simulink model "BuckyWagon_01"  (Simulink 7.5)
settings: Solver=FixedStepDiscrete  StartTime=0.0  StopTime=10.0  RelTol=1e-3
PreLoadFcn:
  | try, eval([bdroot '_setup']); catch, eval('model_setup', ''); end
InitFcn:
  | try, eval([bdroot '_setup']); catch, eval('model_setup', ''); end
undefined symbols (not defined in the file): ECU565, High, Low, miniviewSetup, motohawk_build_version, motohawk_get_faults, motohawk_setup_toolchains, motohawk_trunc_name, motohawk_vardec_config_group, motohawk_vardec_path, tc, True
libraries: MotoHawk_lib x499, simulink x29, motohawk_engine_lib x19, miniview_lib x10, motohawk_control_primitives_lib x8, motohawk_annotations_lib x2
(part 7 of 9)

== system BuckyWagon_01/Strategy/MiniViewDisplay/GetFaultName ==
  Chart : Stateflow chart  TreatAsAtomicUnit=on
  Fault Iterator : Subsystem  TreatAsAtomicUnit=on
  Unit Delay : UnitDelay  SampleTime=-1
  Unit Delay1 : UnitDelay  SampleTime=-1
  getStringLength : Stateflow chart  TreatAsAtomicUnit=on
  motohawk_calibration : MotoHawk_lib/Calibration & Probing Blocks/motohawk_calibration  nam='DisplayFaults'  val=0  storage=Calibration  show_more=on  name_source=Use Parameter  data_type=boolean  read_level=1  write_level=1  ovr_cals=on  view_as=Enumeration  enum_struct={'Disabled', 'Enabled'}  vector_style=Wide Row  use_help_units=on  help='Enable displaying faults when they are active.'  units=''  use_header_enum=off  row_header_enum={}  col_header_enum={}  use_min_max=off  min_val=-inf  max_val=inf  use_precision=off  precision=''  gain=1  offset=0  exp=1  use_mototune_group=off  mototune_group=motohawk_vardec_path(gcb)
  motohawk_calibration1 : MotoHawk_lib/Calibration & Probing Blocks/motohawk_calibration  nam='InvertMode'  val=0  storage=Calibration  show_more=on  name_source=Use Parameter  data_type=boolean  read_level=1  write_level=1  ovr_cals=on  view_as=Enumeration  enum_struct={'Normal', 'Inverted'}  vector_style=Wide Row  use_help_units=on  help='Sets the background color for the text.'  units=''  use_header_enum=off  row_header_enum={}  col_header_enum={}  use_min_max=off  min_val=-inf  max_val=inf  use_precision=off  precision=''  gain=1  offset=0  exp=1  use_mototune_group=off  mototune_group=motohawk_vardec_path(gcb)
  motohawk_calibration2 : MotoHawk_lib/Calibration & Probing Blocks/motohawk_calibration  nam='noErrText'  val=[uint8(' BuckEV') 0 0 0]  storage=Calibration  show_more=on  name_source=Use Parameter  data_type=uint8  read_level=1  write_level=1  ovr_cals=on  view_as=Text  enum_struct={'Disabled', 'Enabled'}  vector_style=Wide Row  use_help_units=on  help='Text to display if there are no faults.'  units=''  use_header_enum=off  row_header_enum={}  col_header_enum={}  use_min_max=off  min_val=-inf  max_val=inf  use_precision=off  precision=''  gain=1  offset=0  exp=1  use_mototune_group=off  mototune_group=motohawk_vardec_path(gcb)
  motohawk_calibration3 : MotoHawk_lib/Calibration & Probing Blocks/motohawk_calibration  nam='dispLength'  val=7  storage=Calibration  show_more=on  name_source=Use Parameter  data_type=uint8  read_level=1  write_level=1  ovr_cals=on  view_as=Number  enum_struct={'Disabled', 'Enabled'}  vector_style=Wide Row  use_help_units=on  help='Number of characters to display when scrolling fault name.'  units=''  use_header_enum=off  row_header_enum={}  col_header_enum={}  use_min_max=on  min_val=0  max_val=9  use_precision=on  precision=''  gain=1  offset=0  exp=1  use_mototune_group=off  mototune_group=motohawk_vardec_path(gcb)
  motohawk_calibration4 : MotoHawk_lib/Calibration & Probing Blocks/motohawk_calibration  nam='lastScrollTime'  val=1/0.005  storage=Calibration  show_more=on  name_source=Use Parameter  data_type=uint16  read_level=1  write_level=1  ovr_cals=on  view_as=Number  enum_struct={'Disabled', 'Enabled'}  vector_style=Wide Row  use_help_units=on  help='Time to spend on the last view of the scroll'  units='s'  use_header_enum=off  row_header_enum={}  col_header_enum={}  use_min_max=on  min_val=0  max_val=5  use_precision=on  precision='1.3'  gain=0.005  offset=0  exp=1  use_mototune_group=off  mototune_group=motohawk_vardec_path(gcb)
  motohawk_calibration5 : MotoHawk_lib/Calibration & Probing Blocks/motohawk_calibration  nam='scrollTime'  val=0.6/0.005  storage=Calibration  show_more=on  name_source=Use Parameter  data_type=uint16  read_level=1  write_level=1  ovr_cals=on  view_as=Number  enum_struct={'Disabled', 'Enabled'}  vector_style=Wide Row  use_help_units=on  help='Time to spend on each view of the scroll'  units='s'  use_header_enum=off  row_header_enum={}  col_header_enum={}  use_min_max=on  min_val=0  max_val=5  use_precision=on  precision='1.3'  gain=0.005  offset=0  exp=1  use_mototune_group=off  mototune_group=motohawk_vardec_path(gcb)
  motohawk_calibration6 : MotoHawk_lib/Calibration & Probing Blocks/motohawk_calibration  nam='minTime'  val=3/0.005  storage=Calibration  show_more=on  name_source=Use Parameter  data_type=uint16  read_level=1  write_level=1  ovr_cals=on  view_as=Number  enum_struct={'Disabled', 'Enabled'}  vector_style=Wide Row  use_help_units=on  help='Minimum time to display each fault name.'  units='s'  use_header_enum=off  row_header_enum={}  col_header_enum={}  use_min_max=on  min_val=0  max_val=5  use_precision=on  precision='1.3'  gain=0.005  offset=0  exp=1  use_mototune_group=off  mototune_group=motohawk_vardec_path(gcb)
  motohawk_calibration7 : MotoHawk_lib/Calibration & Probing Blocks/motohawk_calibration  nam='firstScrollTime'  val=1/0.005  storage=Calibration  show_more=on  name_source=Use Parameter  data_type=uint16  read_level=1  write_level=1  ovr_cals=on  view_as=Number  enum_struct={'Disabled', 'Enabled'}  vector_style=Wide Row  use_help_units=on  help='Time to spend on first view of the scroll'  units='s'  use_header_enum=off  row_header_enum={}  col_header_enum={}  use_min_max=on  min_val=0  max_val=5  use_precision=on  precision='1.3'  gain=0.005  offset=0  exp=1  use_mototune_group=off  mototune_group=motohawk_vardec_path(gcb)
  motohawk_probe : MotoHawk_lib/Calibration & Probing Blocks/motohawk_probe  nam='minTimer'  show_more=on  name_source=Use Parameter  read_level=1  view_as=Number  enum_struct={'Disabled', 'Enabled'}  vector_style=Wide Row  use_help_units=off  help=''  units=''  use_header_enum=off  row_header_enum={}  col_header_enum={}  use_precision=on  precision='1.3'  gain=0.005  offset=0  exp=1  use_mototune_group=off  mototune_group=motohawk_vardec_path(gcb)
  motohawk_probe2 : MotoHawk_lib/Calibration & Probing Blocks/motohawk_probe  nam='scrollTimer'  show_more=on  name_source=Use Parameter  read_level=1  view_as=Number  enum_struct={'Disabled', 'Enabled'}  vector_style=Wide Row  use_help_units=off  help=''  units=''  use_header_enum=off  row_header_enum={}  col_header_enum={}  use_precision=on  precision='1.3'  gain=0.005  offset=0  exp=1  use_mototune_group=off  mototune_group=motohawk_vardec_path(gcb)
  motohawk_probe3 : MotoHawk_lib/Calibration & Probing Blocks/motohawk_probe  nam='scrollIndex'  show_more=off  name_source=Use Parameter  read_level=1  view_as=Number  enum_struct={'Disabled', 'Enabled'}  vector_style=Wide Row  use_help_units=off  help=''  units=''  use_header_enum=off  row_header_enum={}  col_header_enum={}  use_precision=off  precision=''  gain=1  offset=0  exp=1  use_mototune_group=off  mototune_group=motohawk_vardec_path(gcb)
  Name : Outport  OutDataType=sfix(16)  OutScaling=2^0
  Mode : Outport  Port=2  OutDataType=sfix(16)  OutScaling=2^0
  wires:
  Chart/6(getNewFault) -> Fault Iterator/Trigger
  Chart/2(text) -> Name/1
  Chart/1(mode) -> Mode/1
  Chart/3(minTimer) -> motohawk_probe/1
  Chart/4(scrollIndex) -> motohawk_probe3/1
  Chart/5(scrollTimer) -> motohawk_probe2/1
  motohawk_calibration/1 -> Chart/7(dispFaults)
  motohawk_calibration1/1 -> Chart/1(invertMode)
  motohawk_calibration2/1 -> Chart/2(noErrText)
  motohawk_calibration3/1 -> Chart/3(dispLength)
  Fault Iterator/2(valid) -> Unit Delay1/1
  Fault Iterator/1(Name) -> Unit Delay/1
  motohawk_calibration4/1 -> Chart/4(lastScrollTime)
  motohawk_calibration5/1 -> Chart/5(scrollTime)
  motohawk_calibration6/1 -> Chart/8(minTime)
  getStringLength/1(faultNameLength) -> Chart/9(faultNameLen)
  Unit Delay/1 -> Chart/10(faultName), getStringLength/1(faultName)
  Unit Delay1/1 -> Chart/11(faultValid)
  motohawk_calibration7/1 -> Chart/6(firstScrollTime)

== system BuckyWagon_01/Strategy/MiniViewDisplay/Menu Button ==
  CAN Receive Slot Trigger : MotoHawk_lib/CAN Blocks/CAN Receive Slot Trigger  Tag=Trigger  slot='miniview_button_menu'  inherited=on  function_name=Trigger_CAN_Slot_miniview_button_menu_2154p0004
  Demux : Demux  Outputs=2
  Subsystem : Subsystem
  Update : Outport  OutDataType=sfix(16)  OutScaling=2^0
  Menu Asserted : Outport  Port=2  OutDataType=sfix(16)  OutScaling=2^0
  Menu Count : Outport  Port=3  OutDataType=sfix(16)  OutScaling=2^0
  wires:
  Subsystem/1(Out1) -> Menu Asserted/1
  Demux/1 -> Subsystem/Trigger
  CAN Receive Slot Trigger/1 -> Demux/1
  Demux/2 -> Update/1
  Subsystem/2(Out2) -> Menu Count/1

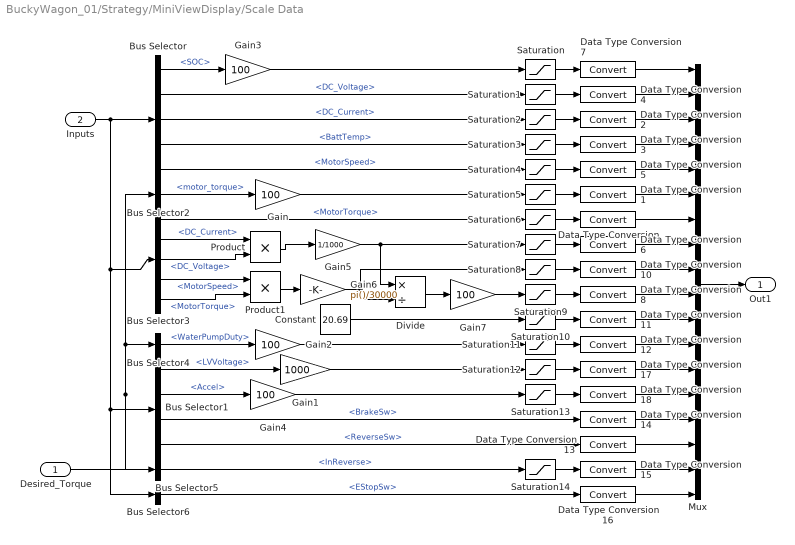
== system BuckyWagon_01/Strategy/MiniViewDisplay/Scale Data ==
  Desired_Torque : Inport  OutDataType=sfix(16)  OutScaling=2^0
  Inputs : Inport  Port=2  OutDataType=sfix(16)  OutScaling=2^0
  Bus Selector : BusSelector  OutputSignals=Virtual.SOC,Physical.DC_Voltage,Physical.DC_Current,Physical.BattTemp,Physical.MotorSpeed
  Bus Selector1 : BusSelector  OutputSignals=Physical.LVVoltage,Physical.Accel,Physical.BrakeSw,Physical.ReverseSw
  Bus Selector2 : BusSelector  OutputSignals=motor_torque
  Bus Selector3 : BusSelector  OutputSignals=Physical.MotorTorque,Physical.DC_Current,Physical.DC_Voltage,Physical.MotorSpeed,Physical.MotorTorque
  Bus Selector4 : BusSelector  OutputSignals=WaterPumpDuty
  Bus Selector5 : BusSelector  OutputSignals=InReverse
  Bus Selector6 : BusSelector  OutputSignals=Physical.EStopSw
  Constant : Constant  Value=20.69  OutDataType=fixdt(1, 16)  OutScaling=2^0
  Data Type Conversion{,1..8,10..18} (18 alike) : DataTypeConversion  OutDataType=sfix(16)  OutScaling=2^0
  Divide : Product  Inputs=*/  OutDataType=sfix(16)  OutScaling=2^-10
  Gain{,2..4,7} (5 alike) : Gain  Gain=100  ParameterDataType=sfix(16)  ParameterScaling=2^0  OutDataType=sfix(16)  OutScaling=2^0  OutDataTypeStr=Inherit: Inherit via back propagation
  Gain1 : Gain  Gain=1000  ParameterDataType=sfix(16)  ParameterScaling=2^0  OutDataType=sfix(16)  OutScaling=2^0  OutDataTypeStr=Inherit: Inherit via back propagation
  Gain5 : Gain  Gain=1/1000  ParameterDataType=sfix(16)  ParameterScaling=2^0  OutDataType=sfix(16)  OutScaling=2^0  OutDataTypeStr=Inherit: Inherit via back propagation
  Gain6 : Gain  Gain=pi()/30000  ParameterDataType=sfix(16)  ParameterScaling=2^0  OutDataType=sfix(16)  OutScaling=2^0  OutDataTypeStr=Inherit: Inherit via back propagation
  Mux : Mux  Inputs=18
  Product : Product  OutDataType=sfix(16)  OutScaling=2^0  RndMeth=Zero
  Product1 : Product  OutDataType=sfix(16)  OutScaling=2^0  RndMeth=Zero
  Saturation{,1..8,10..14} (14 alike) : Saturate  UpperLimit=32767  LowerLimit=-32767  OutDataType=sfix(16)  OutScaling=2^0
  Saturation9 : Saturate  UpperLimit=100  LowerLimit=0  OutDataType=sfix(16)  OutScaling=2^0
  Out1 : Outport  OutDataType=sfix(16)  OutScaling=2^0
  wires:
  Desired_Torque/1 -> Bus Selector2/1, Bus Selector4/1, Bus Selector5/1
  Bus Selector/3 -> Saturation2/1  "<DC_Current>"
  Bus Selector/4 -> Saturation3/1  "<BattTemp>"
  Bus Selector/2 -> Saturation1/1  "<DC_Voltage>"
  Bus Selector/5 -> Saturation4/1  "<MotorSpeed>"
  Bus Selector/1 -> Gain3/1  "<SOC>"
  Mux/1 -> Out1/1
  Gain3/1 -> Saturation/1
  Data Type Conversion4/1 -> Mux/2
  Data Type Conversion2/1 -> Mux/3
  Data Type Conversion3/1 -> Mux/4
  Data Type Conversion5/1 -> Mux/5
  Gain/1 -> Saturation5/1
  Bus Selector2/1 -> Gain/1  "<motor_torque>"
  Inputs/1 -> Bus Selector/1, Bus Selector3/1, Bus Selector1/1, Bus Selector6/1
  Bus Selector3/1 -> Saturation6/1  "<MotorTorque>"
  Bus Selector3/2 -> Product/1  "<DC_Current>"
  Bus Selector3/3 -> Product/2  "<DC_Voltage>"
  Product/1 -> Gain5/1
  Bus Selector3/4 -> Product1/1  "<MotorSpeed>"
  Bus Selector3/5 -> Product1/2  "<MotorTorque>"
  Product1/1 -> Gain6/1
  Constant/1 -> Saturation10/1
  Gain5/1 -> Divide/1, Saturation7/1
  Gain6/1 -> Divide/2, Saturation8/1
  Data Type Conversion/1 -> Mux/7
  Divide/1 -> Gain7/1
  Gain7/1 -> Saturation9/1
  Data Type Conversion6/1 -> Mux/8
  Data Type Conversion10/1 -> Mux/9
  Bus Selector4/1 -> Gain2/1  "<WaterPumpDuty>"
  Gain2/1 -> Saturation11/1
  Bus Selector1/1 -> Gain1/1  "<LVVoltage>"
  Bus Selector1/2 -> Gain4/1  "<Accel>"
  Bus Selector1/3 -> Data Type Conversion14/1  "<BrakeSw>"
  Bus Selector1/4 -> Data Type Conversion13/1  "<ReverseSw>"
  Gain1/1 -> Saturation12/1
  Gain4/1 -> Saturation13/1
  Data Type Conversion14/1 -> Mux/15
  Data Type Conversion13/1 -> Mux/16
  Bus Selector5/1 -> Saturation14/1  "<InReverse>"
  Data Type Conversion15/1 -> Mux/17
  Bus Selector6/1 -> Data Type Conversion16/1  "<EStopSw>"
  Data Type Conversion16/1 -> Mux/18
  Data Type Conversion1/1 -> Mux/6
  Data Type Conversion7/1 -> Mux/1
  Data Type Conversion8/1 -> Mux/10
  Data Type Conversion11/1 -> Mux/11
  Data Type Conversion12/1 -> Mux/12
  Data Type Conversion17/1 -> Mux/13
  Data Type Conversion18/1 -> Mux/14
  Saturation/1 -> Data Type Conversion7/1
  Saturation1/1 -> Data Type Conversion4/1
  Saturation2/1 -> Data Type Conversion2/1
  Saturation3/1 -> Data Type Conversion3/1
  Saturation4/1 -> Data Type Conversion5/1
  Saturation5/1 -> Data Type Conversion1/1
  Saturation6/1 -> Data Type Conversion/1
  Saturation7/1 -> Data Type Conversion6/1
  Saturation8/1 -> Data Type Conversion10/1
  Saturation9/1 -> Data Type Conversion8/1
  Saturation10/1 -> Data Type Conversion11/1
  Saturation11/1 -> Data Type Conversion12/1
  Saturation12/1 -> Data Type Conversion17/1
  Saturation13/1 -> Data Type Conversion18/1
  Saturation14/1 -> Data Type Conversion15/1

== system BuckyWagon_01/Strategy/MiniViewDisplay/Send String_efficient ==
  string # : Inport  OutDataType=sfix(16)  OutScaling=2^0
  string : Inport  Port=2  OutDataType=sfix(16)  OutScaling=2^0
  Trigger : TriggerPort  TriggerType=function-call
  Demux : Demux  Outputs=2
  Function-Call Generator : simulink/Ports & Subsystems/Function-Call Generator  sample_time=-1  numberOfIterations=1
  Signal Specification : SignalSpecification  Dimensions=18  DataType=uint8  OutDataType=sfix(16)  OutScaling=2^0  OutDataTypeStr=uint8
  Subsystem : Subsystem
  Next : Outport  OutDataType=sfix(16)  OutScaling=2^0
  wires:
  Signal Specification/1 -> Subsystem/2(string)
  Demux/2 -> Next/1
  Function-Call Generator/1 -> Demux/1
  Demux/1 -> Subsystem/Trigger
  string/1 -> Signal Specification/1  "b0"
  string #/1 -> Subsystem/1(string #)  "string"

== system BuckyWagon_01/Strategy/MiniViewDisplay/Up Button ==
  CAN Receive Slot Trigger : MotoHawk_lib/CAN Blocks/CAN Receive Slot Trigger  Tag=Trigger  slot='miniview_button_up'  inherited=on  function_name=Trigger_CAN_Slot_miniview_button_up_2402p0004
  Demux : Demux  Outputs=2
  Subsystem : Subsystem
  Update : Outport  OutDataType=sfix(16)  OutScaling=2^0
  Up Asserted : Outport  Port=2  OutDataType=sfix(16)  OutScaling=2^0
  Up Count : Outport  Port=3  OutDataType=sfix(16)  OutScaling=2^0
  wires:
  Subsystem/2(Up Count) -> Up Count/1
  Demux/2 -> Update/1
  CAN Receive Slot Trigger/1 -> Demux/1
  Demux/1 -> Subsystem/Trigger
  Subsystem/1(Up Asserted) -> Up Asserted/1

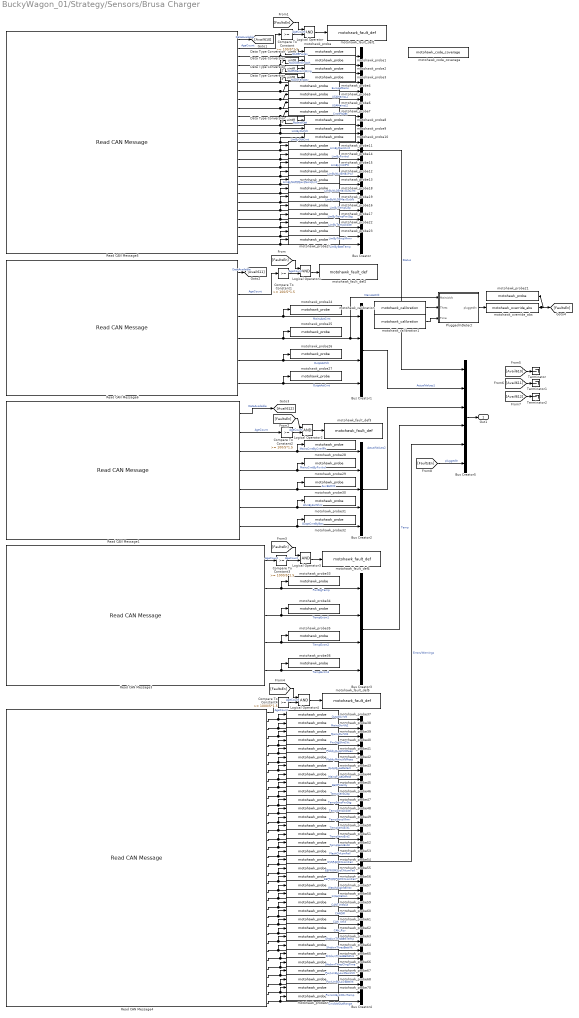
== system BuckyWagon_01/Strategy/Sensors/Brusa Charger ==
  Bus Creator : BusCreator  Inputs=23
  Bus Creator1 : BusCreator
  Bus Creator2 : BusCreator  Inputs=5
  Bus Creator3 : BusCreator
  Bus Creator4 : BusCreator  Inputs=34
  Bus Creator5 : BusCreator  Inputs=6
  Compare To Constant : simulink/Logic and Bit Operations/Compare To Constant  SystemSampleTime=-1  relop=>=  const=100/5*1.5  LogicOutDataTypeMode=boolean  ZeroCross=off
  Compare To Constant1 : simulink/Logic and Bit Operations/Compare To Constant  SystemSampleTime=-1  relop=>=  const=100/5*1.5  LogicOutDataTypeMode=boolean  ZeroCross=off
  Compare To Constant2 : simulink/Logic and Bit Operations/Compare To Constant  SystemSampleTime=-1  relop=>=  const=100/5*1.5  LogicOutDataTypeMode=boolean  ZeroCross=off
  Compare To Constant3 : simulink/Logic and Bit Operations/Compare To Constant  SystemSampleTime=-1  relop=>=  const=1000/5*1.5  LogicOutDataTypeMode=boolean  ZeroCross=off
  Compare To Constant4 : simulink/Logic and Bit Operations/Compare To Constant  SystemSampleTime=-1  relop=>=  const=1000/5*1.5  LogicOutDataTypeMode=boolean  ZeroCross=off
  Data Type Conversion{,1..4} (5 alike) : DataTypeConversion  OutDataTypeMode=uint8  OutDataType=sfix(16)  OutScaling=2^0  OutDataTypeStr=uint8
  Logical Operator{,1..4} (5 alike) : Logic  AllPortsSameDT=off  OutDataTypeMode=boolean  OutDataTypeStr=boolean
  PluggedInDetect : Subsystem
  Read CAN Message1 : MotoHawk_lib/CAN Blocks/Read CAN Message  nam=['CAN_' num2str(1)]  bus=-2  msg=can_BRUSA_612  queue=1  slot=''  valid=on  stale=on  labelwires=on
  Read CAN Message3 : MotoHawk_lib/CAN Blocks/Read CAN Message  nam=['CAN_' num2str(1)]  bus=-2  msg=can_BRUSA_613  queue=1  slot=''  valid=off  stale=on  labelwires=on
  Read CAN Message4 : MotoHawk_lib/CAN Blocks/Read CAN Message  nam=['CAN_' num2str(1)]  bus=-2  msg=can_BRUSA_614  queue=1  slot=''  valid=off  stale=on  labelwires=on
  Read CAN Message5 : MotoHawk_lib/CAN Blocks/Read CAN Message  nam=['CAN_' num2str(1)]  bus=-2  msg=can_BRUSA_610  queue=1  slot=''  valid=on  stale=on  labelwires=on
  Read CAN Message6 : MotoHawk_lib/CAN Blocks/Read CAN Message  nam=['CAN_' num2str(1)]  bus=-2  msg=can_BRUSA_611  queue=1  slot=''  valid=on  stale=on  labelwires=on
  Terminator : Terminator
  Terminator1 : Terminator
  Terminator2 : Terminator
  motohawk_calibration : MotoHawk_lib/Calibration & Probing Blocks/motohawk_calibration  nam='PluggedInMainsThes'  val=90  storage=Calibration  show_more=on  name_source=Use Parameter  data_type=Inherit from 'Default Value'  read_level=1  write_level=1  ovr_cals=on  view_as=Number  enum_struct={'Disabled', 'Enabled'}  vector_style=Wide Row  use_help_units=on  help='Above this mains voltage the charger is plugged in.'  units='V'  use_header_enum=off  row_header_enum={}  col_header_enum={}  use_min_max=off  min_val=-inf  max_val=inf  use_precision=off  precision=''  gain=1  offset=0  exp=1  use_mototune_group=off  mototune_group=motohawk_vardec_path(gcb)
  motohawk_calibration1 : MotoHawk_lib/Calibration & Probing Blocks/motohawk_calibration  nam='PluggedInHistTime'  val=0.5/0.005  storage=Calibration  show_more=on  name_source=Use Parameter  data_type=Inherit from 'Default Value'  read_level=1  write_level=1  ovr_cals=on  view_as=Number  enum_struct={'Disabled', 'Enabled'}  vector_style=Wide Row  use_help_units=on  help='Historesis time for plugged in detection.'  units='s'  use_header_enum=off  row_header_enum={}  col_header_enum={}  use_min_max=off  min_val=-inf  max_val=inf  use_precision=on  precision='1.2'  gain=0.005  offset=0  exp=1  use_mototune_group=off  mototune_group=motohawk_vardec_path(gcb)
  motohawk_code_coverage : MotoHawk_lib/Extra Development Blocks/motohawk_code_coverage
  motohawk_fault_def1 : MotoHawk_lib/Fault Management Blocks/motohawk_fault_def  nam='canNLG5_610'  mode=Enabled  id=[]  x=100/5*0.5  y=100/5*2  input_suspected=on  indeterminate=off  increment_xy=on  downsample_count=1  ovr_cals=on  ovr_actions=on  show_actions=on  action1_name='Charge_Fault'  action1_cond=Active  action2_name=''  action2_cond=(None)  action3_name=''  action3_cond=(None)  action4_name=''  action4_cond=(None)
  motohawk_fault_def2 : MotoHawk_lib/Fault Management Blocks/motohawk_fault_def  nam='canNLG5_611'  mode=Enabled  id=[]  x=100/5*0.5  y=100/5*2  input_suspected=on  indeterminate=off  increment_xy=on  downsample_count=1  ovr_cals=on  ovr_actions=on  show_actions=on  action1_name='Charge_Fault'  action1_cond=Active  action2_name=''  action2_cond=(None)  action3_name=''  action3_cond=(None)  action4_name=''  action4_cond=(None)
  motohawk_fault_def3 : MotoHawk_lib/Fault Management Blocks/motohawk_fault_def  nam='canNLG5_612'  mode=Enabled  id=[]  x=100/5*0.5  y=100/5*2  input_suspected=on  indeterminate=off  increment_xy=on  downsample_count=1  ovr_cals=on  ovr_actions=on  show_actions=on  action1_name='Charge_Fault'  action1_cond=(None)  action2_name=''  action2_cond=(None)  action3_name=''  action3_cond=(None)  action4_name=''  action4_cond=(None)
  motohawk_fault_def4 : MotoHawk_lib/Fault Management Blocks/motohawk_fault_def  nam='canNLG5_613'  mode=Enabled  id=[]  x=1000/5*0.5  y=1000/5*2  input_suspected=on  indeterminate=off  increment_xy=on  downsample_count=1  ovr_cals=on  ovr_actions=on  show_actions=off  action1_name=''  action1_cond=(None)  action2_name=''  action2_cond=(None)  action3_name=''  action3_cond=(None)  action4_name=''  action4_cond=(None)
  motohawk_fault_def5 : MotoHawk_lib/Fault Management Blocks/motohawk_fault_def  nam='canNLG5_614'  mode=Enabled  id=[]  x=1000/5*0.5  y=1000/5*2  input_suspected=on  indeterminate=off  increment_xy=on  downsample_count=1  ovr_cals=on  ovr_actions=on  show_actions=off  action1_name=''  action1_cond=(None)  action2_name=''  action2_cond=(None)  action3_name=''  action3_cond=(None)  action4_name=''  action4_cond=(None)
  motohawk_override_abs : MotoHawk_lib/Calibration & Probing Blocks/motohawk_override_abs  SystemSampleTime=-1  parent_name='pluggedIn'  parent_val=0  show_more=off  name_source=Use Parameter  parent_read_level=1  parent_override_level=1  view_as=Number  enum_struct={'Disabled', 'Enabled'}  use_help_units=off  parent_help=''  parent_units=''  use_min_max=off  parent_min=-inf  parent_max=inf  use_precision=off  parent_precision=''  parent_gain=1  parent_offset=0  parent_exp=1  use_mototune_group=off  parent_group=motohawk_vardec_path(gcb)
  motohawk_probe : MotoHawk_lib/Calibration & Probing Blocks/motohawk_probe  nam='NLG5PwrEn'  show_more=on  name_source=Use Parameter  read_level=1  view_as=Enumeration  enum_struct={'Disabled', 'Enabled'}  vector_style=Wide Row  use_help_units=off  help=''  units=''  use_header_enum=off  row_header_enum={}  col_header_enum={}  use_precision=off  precision=''  gain=1  offset=0  exp=1  use_mototune_group=off  mototune_group=motohawk_vardec_path(gcb)
  motohawk_probe1 : MotoHawk_lib/Calibration & Probing Blocks/motohawk_probe  nam='NLG5GenErrLtch'  show_more=on  name_source=Use Parameter  read_level=1  view_as=Enumeration  enum_struct={'No Error', 'ERROR'}  vector_style=Wide Row  use_help_units=off  help=''  units=''  use_header_enum=off  row_header_enum={}  col_header_enum={}  use_precision=off  precision=''  gain=1  offset=0  exp=1  use_mototune_group=off  mototune_group=motohawk_vardec_path(gcb)
  motohawk_probe{4..7,9..20,22..70} (65 alike) : MotoHawk_lib/Calibration & Probing Blocks/motohawk_probe  nam='Probe'  show_more=on  name_source=Use Input Wire Name  read_level=1  view_as=Number  enum_struct={'Disabled', 'Enabled'}  vector_style=Wide Row  use_help_units=off  help=''  units=''  use_header_enum=off  row_header_enum={}  col_header_enum={}  use_precision=off  precision=''  gain=1  offset=0  exp=1  use_mototune_group=off  mototune_group=motohawk_vardec_path(gcb)
  motohawk_probe2 : MotoHawk_lib/Calibration & Probing Blocks/motohawk_probe  nam='NLG5GenLimWrng'  show_more=on  name_source=Use Parameter  read_level=1  view_as=Enumeration  enum_struct={'No Warn', 'WARNING'}  vector_style=Wide Row  use_help_units=off  help=''  units=''  use_header_enum=off  row_header_enum={}  col_header_enum={}  use_precision=off  precision=''  gain=1  offset=0  exp=1  use_mototune_group=off  mototune_group=motohawk_vardec_path(gcb)
  motohawk_probe21 : MotoHawk_lib/Calibration & Probing Blocks/motohawk_probe  nam='pluggedIn'  show_more=off  name_source=Use Parameter  read_level=1  view_as=Number  enum_struct={'Disabled', 'Enabled'}  vector_style=Wide Row  use_help_units=off  help=''  units=''  use_header_enum=off  row_header_enum={}  col_header_enum={}  use_precision=off  precision=''  gain=1  offset=0  exp=1  use_mototune_group=off  mototune_group=motohawk_vardec_path(gcb)
  motohawk_probe3 : MotoHawk_lib/Calibration & Probing Blocks/motohawk_probe  nam='NLG5FanActv'  show_more=on  name_source=Use Parameter  read_level=1  view_as=Enumeration  enum_struct={'Off', 'On'}  vector_style=Wide Row  use_help_units=off  help=''  units=''  use_header_enum=off  row_header_enum={}  col_header_enum={}  use_precision=off  precision=''  gain=1  offset=0  exp=1  use_mototune_group=off  mototune_group=motohawk_vardec_path(gcb)
  motohawk_probe8 : MotoHawk_lib/Calibration & Probing Blocks/motohawk_probe  nam='BypassDet'  show_more=on  name_source=Use Parameter  read_level=1  view_as=Enumeration  enum_struct={'none', 'DC', 'AC in Phase', 'AC not in Phase'}  vector_style=Wide Row  use_help_units=off  help=''  units=''  use_header_enum=off  row_header_enum={}  col_header_enum={}  use_precision=off  precision=''  gain=1  offset=0  exp=1  use_mototune_group=off  mototune_group=motohawk_vardec_path(gcb)
  Out1 : Outport  OutDataType=sfix(16)  OutScaling=2^0
  wires:
  Read CAN Message5/2 -> Compare To Constant/1  "AgeCount"
  Read CAN Message5/3 -> Bus Creator/1, Data Type Conversion/1  "NLG5PwrEn"
  Read CAN Message5/4 -> Bus Creator/2, Data Type Conversion1/1  "NLG5GenErrLtch"
  Read CAN Message5/5 -> Bus Creator/3, Data Type Conversion2/1  "NLG5GenLimWrng"
  Read CAN Message5/6 -> Bus Creator/4, Data Type Conversion3/1  "NLG5FanActv"
  Read CAN Message5/7 -> Bus Creator/5, motohawk_probe4/1  "EuropeMains"
  Read CAN Message5/8 -> Bus Creator/6, motohawk_probe5/1  "USAMainsL1"
  Read CAN Message5/9 -> Bus Creator/7, motohawk_probe6/1  "USAMainsL2"
  Read CAN Message5/10 -> Bus Creator/8, motohawk_probe7/1  "CntrlPltDet"
  Read CAN Message5/11 -> Bus Creator/9, Data Type Conversion4/1  "BypassDet"
  Read CAN Message5/12 -> Bus Creator/10, motohawk_probe9/1  "LimByOutVlt"
  Read CAN Message5/13 -> Bus Creator/11, motohawk_probe10/1  "LimByOutCrnt"
  Read CAN Message5/14 -> Bus Creator/12, motohawk_probe11/1  "LimByMainCrnt"
  Read CAN Message5/15 -> Bus Creator/13, motohawk_probe14/1  "LimByPwrInd"
  Read CAN Message5/16 -> Bus Creator/14, motohawk_probe15/1  "LimByCntrlPlt"
  Read CAN Message5/17 -> Bus Creator/15, motohawk_probe12/1  "LimByNLG5MaxPwr"
  Read CAN Message5/18 -> Bus Creator/16, motohawk_probe13/1  "LimByNLG5MaxMainsCrnt"
  Read CAN Message5/19 -> Bus Creator/17, motohawk_probe18/1  "LimByNLG5MaxOutCrnt"
  Read CAN Message5/20 -> Bus Creator/18, motohawk_probe19/1  "LimByNLG5MaxOutVlt"
  Read CAN Message5/21 -> Bus Creator/19, motohawk_probe16/1  "LimByTempCap"
  Read CAN Message5/22 -> Bus Creator/20, motohawk_probe17/1  "LimByTempPwrStg"
  Read CAN Message5/23 -> Bus Creator/21, motohawk_probe22/1  "LimByTempDiode"
  Read CAN Message5/24 -> Bus Creator/22, motohawk_probe23/1  "LimByTempXfrmr"
  Read CAN Message5/25 -> Bus Creator/23, motohawk_probe20/1  "LimByBattTemp"
  Read CAN Message1/3 -> motohawk_probe28/1, Bus Creator2/1  "MainsCrntByCntrlPlt"
  Read CAN Message1/4 -> motohawk_probe29/1, Bus Creator2/2  "MainsCrntByPwrInd"
  Read CAN Message1/5 -> motohawk_probe30/1, Bus Creator2/3  "AuxBattVlt"
  Read CAN Message1/6 -> motohawk_probe31/1, Bus Creator2/4  "AhrsByExtShnt"
  Read CAN Message1/7 -> Bus Creator2/5, motohawk_probe32/1  "OutptCrntByBstr"
  Read CAN Message1/2 -> Compare To Constant2/1  "AgeCount"
  Read CAN Message6/3 -> Bus Creator1/1, motohawk_probe24/1  "MainsActCrnt"
  Read CAN Message6/4 -> motohawk_probe25/1, Bus Creator1/2, PluggedInDetect/1(MainsVolt)  "MainsActVlt"
  Read CAN Message6/5 -> Bus Creator1/3, motohawk_probe26/1  "OutptActVlt"
  Read CAN Message6/6 -> Bus Creator1/4, motohawk_probe27/1  "OutptActCrnt"
  Read CAN Message3/1 -> Compare To Constant3/1  "AgeCount"
  Read CAN Message3/2 -> Bus Creator3/1, motohawk_probe33/1  "PwrStgTemp"
  Read CAN Message3/3 -> Bus Creator3/2, motohawk_probe34/1  "TempExtrn1"
  Read CAN Message3/4 -> Bus Creator3/3, motohawk_probe35/1  "TempExtrn2"
  Read CAN Message3/5 -> Bus Creator3/4, motohawk_probe36/1  "TempExtrn3"
  Read CAN Message4/1 -> Compare To Constant4/1  "AgeCount"
  Read CAN Message4/2 -> Bus Creator4/1, motohawk_probe37/1  "OutptOvrVlt"
  Read CAN Message4/3 -> Bus Creator4/2, motohawk_probe38/1  "MainsOvrVlt2"
  Read CAN Message4/4 -> Bus Creator4/3, motohawk_probe39/1  "MainsOvrVlt1"
  Read CAN Message4/5 -> Bus Creator4/4, motohawk_probe40/1  "PwrStgShrtCkt"
  Read CAN Message4/6 -> Bus Creator4/5, motohawk_probe41/1  "PlsbltyOutptVltMeas"
  Read CAN Message4/7 -> Bus Creator4/6, motohawk_probe42/1  "PlsbltyMainsVltMeas"
  Read CAN Message4/8 -> Bus Creator4/7, motohawk_probe43/1  "OutptFuseDefect"
  Read CAN Message4/9 -> Bus Creator4/8, motohawk_probe44/1  "MainsFuseDefect"
  Read CAN Message4/10 -> Bus Creator4/9, motohawk_probe45/1  "BattPolarity"
  Read CAN Message4/11 -> Bus Creator4/10, motohawk_probe46/1  "TempSensCap"
  Read CAN Message4/12 -> Bus Creator4/11, motohawk_probe47/1  "TempSensPwrStg"
  Read CAN Message4/13 -> Bus Creator4/12, motohawk_probe48/1  "TempSensDiode"
  Read CAN Message4/14 -> Bus Creator4/13, motohawk_probe49/1  "TempSensXfrmr"
  Read CAN Message4/15 -> Bus Creator4/14, motohawk_probe50/1  "TempSensExt1"
  Read CAN Message4/16 -> Bus Creator4/15, motohawk_probe51/1  "TempSensExt2"
  Read CAN Message4/17 -> Bus Creator4/16, motohawk_probe52/1  "TempSensExt3"
  Read CAN Message4/18 -> Bus Creator4/17, motohawk_probe53/1  "FlashChksmFail"
  Read CAN Message4/19 -> Bus Creator4/18, motohawk_probe54/1  "NVSRAMChksmFail"
  Read CAN Message4/20 -> Bus Creator4/19, motohawk_probe55/1  "EEPROMSysChksmFail"
  Read CAN Message4/21 -> Bus Creator4/20, motohawk_probe56/1  "EEPROMPOWChksmFail"
  Read CAN Message4/22 -> Bus Creator4/21, motohawk_probe57/1  "WatchdogInternal"
  Read CAN Message4/23 -> Bus Creator4/22, motohawk_probe58/1  "Initialization"
  Read CAN Message4/24 -> Bus Creator4/23, motohawk_probe59/1  "CANTimeout"
  Read CAN Message4/25 -> Bus Creator4/24, motohawk_probe60/1  "CANOff"
  Bus Creator/1 -> Bus Creator5/1  "Status"
  Bus Creator1/1 -> Bus Creator5/2  "ActualValues1"
  Bus Creator2/1 -> Bus Creator5/3  "ActualValues2"
  Bus Creator3/1 -> Bus Creator5/4  "Temp"
  Bus Creator4/1 -> Bus Creator5/5  "Errors/Warnings"
  Bus Creator5/1 -> Out1/1
  Read CAN Message4/26 -> Bus Creator4/25, motohawk_probe61/1  "CAN_Xmit"
  Read CAN Message4/27 -> Bus Creator4/26, motohawk_probe62/1  "CAN_Rcv"
  Read CAN Message4/28 -> Bus Creator4/27, motohawk_probe63/1  "ShtdwnThrsBattTemp"
  Read CAN Message4/29 -> Bus Creator4/28, motohawk_probe64/1  "ShtdwnThresBattVlt"
  Read CAN Message4/30 -> Bus Creator4/29, motohawk_probe65/1  "ShtdwnThresBattAhrs"
  Read CAN Message4/31 -> Bus Creator4/30, motohawk_probe66/1  "ShtdwnThresChrgTime"
  Read CAN Message4/32 -> Bus Creator4/31, motohawk_probe67/1  "PwrLimByLowMainsVlt"
  Read CAN Message4/33 -> Bus Creator4/32, motohawk_probe68/1  "PwrLimByLowBattVlt"
  Read CAN Message4/34 -> Bus Creator4/33, motohawk_probe70/1  "PwrLimByIntOvrTemp"
  Read CAN Message4/35 -> Bus Creator4/34, motohawk_probe69/1  "CmdValOutRange"
  Data Type Conversion/1 -> motohawk_probe/1
  Data Type Conversion1/1 -> motohawk_probe1/1
  Data Type Conversion2/1 -> motohawk_probe2/1
  Data Type Conversion3/1 -> motohawk_probe3/1
  Data Type Conversion4/1 -> motohawk_probe8/1
  [FaultsEn] -> Logical Operator/1
  Compare To Constant/1 -> Logical Operator/2  "AgeCount"
  Logical Operator/1 -> motohawk_fault_def1/1
  [FaultsEn] -> Logical Operator1/1
  Compare To Constant1/1 -> Logical Operator1/2  "AgeCount"
  Logical Operator1/1 -> motohawk_fault_def2/1
  [FaultsEn] -> Logical Operator2/1
  Compare To Constant2/1 -> Logical Operator2/2  "AgeCount"
  Logical Operator2/1 -> motohawk_fault_def3/1
  [FaultsEn] -> Logical Operator3/1
  Compare To Constant3/1 -> Logical Operator3/2  "AgeCount"
  Logical Operator3/1 -> motohawk_fault_def4/1
  [FaultsEn] -> Logical Operator4/1
  Compare To Constant4/1 -> Logical Operator4/2  "AgeCount"
  Logical Operator4/1 -> motohawk_fault_def5/1
  Read CAN Message5/1 -> [Avail610]  "DataAvailable"
  Read CAN Message6/2 -> Compare To Constant1/1  "AgeCount"
  Read CAN Message6/1 -> [Avail611]  "DataAvailable"
  Read CAN Message1/1 -> [Avail612]  "DataAvailable"
  [FaultsEn] -> Bus Creator5/6  "pluggedIn"
  motohawk_calibration/1 -> PluggedInDetect/2(Thres)
  motohawk_calibration1/1 -> PluggedInDetect/3(Time)
  PluggedInDetect/1(pluggedIn) -> motohawk_override_abs/1
  motohawk_override_abs/1 -> [FaultsEn], motohawk_probe21/1
  [Avail610] -> Terminator/1
  [Avail611] -> Terminator1/1
  [Avail612] -> Terminator2/1

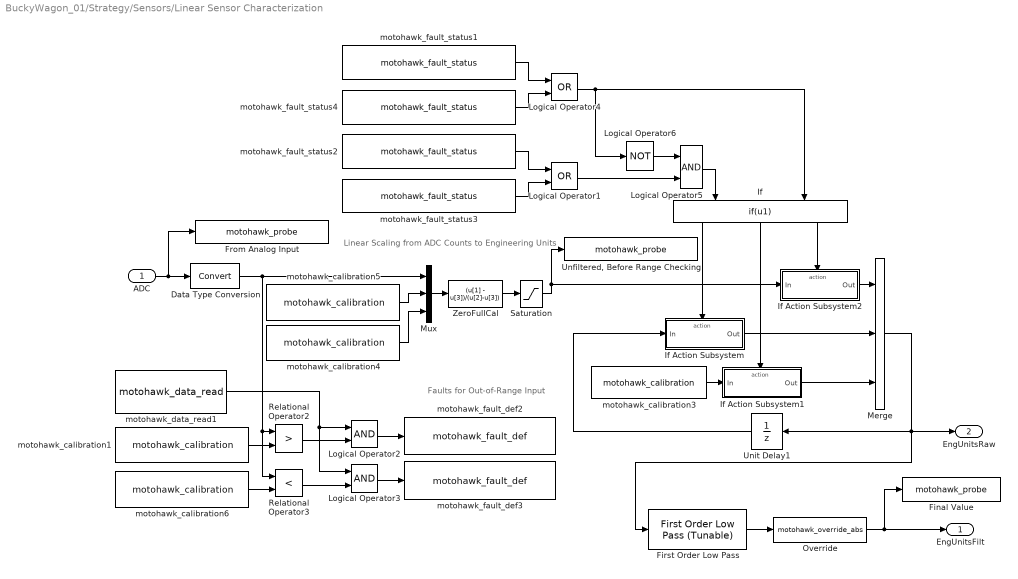
== system BuckyWagon_01/Strategy/Sensors/Linear Sensor Characterization ==
  note: Linear Scaling from ADC Counts
      | to Engineering Units
  note: Faults for
      | Out-of-Range
      | Input
  ADC : Inport  OutDataType=sfix(16)  OutScaling=2^0
  Data Type Conversion : DataTypeConversion  OutDataType=sfix(16)  OutScaling=2^0  SaturateOnIntegerOverflow=on  RndMeth=Zero
  Final Value : MotoHawk_lib/Calibration & Probing Blocks/motohawk_probe  nam=nam  show_more=on  name_source=Use Parameter  read_level=1  view_as=Number  enum_struct={'Disabled', 'Enabled'}  vector_style=Wide Row  use_help_units=on  help='Final value after Linear Sensor Characterization'  units=units  use_header_enum=off  row_header_enum={}  col_header_enum={}  use_precision=off  precision=''  gain=1  offset=0  exp=1  use_mototune_group=on  mototune_group=group
  First Order Low Pass : motohawk_control_primitives_lib/First Order Low Pass (Tunable)  SystemSampleTime=-1  nam=[prefix 'FilterConst']  samp_time=samp_time  group=[group ' | ' nam ' Config']
  From Analog Input : MotoHawk_lib/Calibration & Probing Blocks/motohawk_probe  nam=[prefix 'ADC']  show_more=on  name_source=Use Parameter  read_level=1  view_as=Number  enum_struct={'Disabled', 'Enabled'}  vector_style=Wide Row  use_help_units=on  help='Singal measured directly from sensor'  units=inputunits  use_header_enum=off  row_header_enum={}  col_header_enum={}  use_precision=off  precision=''  gain=1  offset=0  exp=1  use_mototune_group=on  mototune_group=group
  If : If  NumInputs=2  IfExpression=u1  ElseIfExpressions=u2  ZeroCross=off
  If Action Subsystem : Subsystem  TreatAsAtomicUnit=on
      mask Display: disp('Saturate');
  If Action Subsystem1 : Subsystem  TreatAsAtomicUnit=on
      mask Display: disp('Default');
  If Action Subsystem2 : Subsystem  TreatAsAtomicUnit=on
      mask Display: disp('Pass Through');
  Logical Operator1 : Logic  Operator=OR
  Logical Operator2 : Logic
  Logical Operator3 : Logic
  Logical Operator4 : Logic  Operator=OR
  Logical Operator5 : Logic
  Logical Operator6 : Logic  Operator=NOT
  Merge : Merge  Inputs=3
  Mux : Mux  Inputs=3
  Override : MotoHawk_lib/Calibration & Probing Blocks/motohawk_override_abs  SystemSampleTime=-1  parent_name=nam  parent_val=0  show_more=on  name_source=Use Parameter  parent_read_level=1  parent_override_level=1  view_as=Number  enum_struct={'Disabled', 'Enabled'}  use_help_units=on  parent_help='Override result of linear sensor characterization, in engineering units'  parent_units=units  use_min_max=on  parent_min=-inf  parent_max=inf  use_precision=off  parent_precision=''  parent_gain=1  parent_offset=0  parent_exp=1  use_mototune_group=on  parent_group=group
  Relational Operator2 : RelationalOperator  Operator=>  ZeroCross=off  InputSameDT=on
  Relational Operator3 : RelationalOperator  Operator=<  ZeroCross=off  InputSameDT=on
  Saturation : Saturate  UpperLimit=1  LowerLimit=0
  "Unfiltered, Before Range Checking" : MotoHawk_lib/Calibration & Probing Blocks/motohawk_probe  nam=[prefix 'Raw']  show_more=on  name_source=Use Parameter  read_level=1  view_as=Number  enum_struct={'Disabled', 'Enabled'}  vector_style=Wide Row  use_help_units=on  help='After conversion to engineering units, before range checking'  units=units  use_header_enum=off  row_header_enum={}  col_header_enum={}  use_precision=off  precision=''  gain=1  offset=0  exp=1  use_mototune_group=on  mototune_group=group
  Unit Delay1 : UnitDelay  SampleTime=-1
  ZeroFullCal : Fcn  Expr=(u[1] - u[3])/(u[2]-u[3])
  motohawk_calibration1 : MotoHawk_lib/Calibration & Probing Blocks/motohawk_calibration  nam=[prefix 'InputHiFltPos']  val=1020  storage=Calibration  show_more=on  name_source=Use Parameter  data_type=double  read_level=1  write_level=1  ovr_cals=on  view_as=Number  enum_struct={'Disabled', 'Enabled'}  vector_style=Wide Row  use_help_units=on  help='Maximum allowable input, indicating short or open circuit'  units=inputunits  use_header_enum=off  row_header_enum={}  col_header_enum={}  use_min_max=off  min_val=-inf  max_val=inf  use_precision=off  precision=''  gain=1  offset=0  exp=1  use_mototune_group=on  mototune_group=[group ' | ' nam ' Config']
  motohawk_calibration3 : MotoHawk_lib/Calibration & Probing Blocks/motohawk_calibration  nam=[prefix 'DfltValue']  val=1  storage=Calibration  show_more=on  name_source=Use Parameter  data_type=double  read_level=1  write_level=1  ovr_cals=on  view_as=Number  enum_struct={'Disabled', 'Enabled'}  vector_style=Wide Row  use_help_units=on  help="'This is the initial default value should the sensor be in fault on key-up.  Otherwise the sensors outputs the last value prior to faulting'"  units=units  use_header_enum=off  row_header_enum={}  col_header_enum={}  use_min_max=off  min_val=-inf  max_val=inf  use_precision=off  precision=''  gain=1  offset=0  exp=1  use_mototune_group=on  mototune_group=[group ' | ' nam ' Config']
  motohawk_calibration4 : MotoHawk_lib/Calibration & Probing Blocks/motohawk_calibration  nam=[prefix 'Zero']  val=1  storage=Calibration  show_more=on  name_source=Use Parameter  data_type=double  read_level=1  write_level=1  ovr_cals=on  view_as=Number  enum_struct={'Disabled', 'Enabled'}  vector_style=Wide Row  use_help_units=on  help='Scaling from A/D counts to engineering units'  units=[units '/ADC']  use_header_enum=off  row_header_enum={}  col_header_enum={}  use_min_max=off  min_val=-inf  max_val=inf  use_precision=on  precision='5.4'  gain=1  offset=0  exp=1  use_mototune_group=on  mototune_group=[group ' | ' nam ' Config']
  motohawk_calibration5 : MotoHawk_lib/Calibration & Probing Blocks/motohawk_calibration  nam=[prefix 'Full']  val=0  storage=Calibration  show_more=on  name_source=Use Parameter  data_type=double  read_level=1  write_level=1  ovr_cals=on  view_as=Number  enum_struct={'Disabled', 'Enabled'}  vector_style=Wide Row  use_help_units=on  help='Offset after gain in engineering units'  units=units  use_header_enum=off  row_header_enum={}  col_header_enum={}  use_min_max=off  min_val=-inf  max_val=inf  use_precision=off  precision=''  gain=1  offset=0  exp=1  use_mototune_group=on  mototune_group=[group ' | ' nam ' Config']
  motohawk_calibration6 : MotoHawk_lib/Calibration & Probing Blocks/motohawk_calibration  nam=[prefix 'InputLoFltPos']  val=10  storage=Calibration  show_more=on  name_source=Use Parameter  data_type=double  read_level=1  write_level=1  ovr_cals=on  view_as=Number  enum_struct={'Disabled', 'Enabled'}  vector_style=Wide Row  use_help_units=on  help='Minimum allowable input, indicating short or open circuit'  units=inputunits  use_header_enum=off  row_header_enum={}  col_header_enum={}  use_min_max=off  min_val=-inf  max_val=inf  use_precision=off  precision=''  gain=1  offset=0  exp=1  use_mototune_group=on  mototune_group=[group ' | ' nam ' Config']
  motohawk_data_read1 : MotoHawk_lib/Data Storage Blocks/motohawk_data_read  source=Lookup By Name  structure=Scalar  operation=Read entire data structure at once  sz_vec=4  sz_row=2  sz_col=3  typ=boolean  nam='MPRD'  checkNull=on  struct_inst_name='Struct1'  struct_nam='MyStruct'
  motohawk_fault_def2 : MotoHawk_lib/Fault Management Blocks/motohawk_fault_def  nam=[prefix 'RangeHigh']  mode=Enabled  id=[]  x=25  y=50  input_suspected=on  indeterminate=off  increment_xy=on  downsample_count=1  ovr_cals=on  ovr_actions=on  show_actions=off  action1_name=''  action1_cond=(None)  action2_name=''  action2_cond=(None)  action3_name=''  action3_cond=(None)  action4_name=''  action4_cond=(None)
  motohawk_fault_def3 : MotoHawk_lib/Fault Management Blocks/motohawk_fault_def  nam=[prefix 'RangeLow']  mode=Enabled  id=[]  x=25  y=50  input_suspected=on  indeterminate=off  increment_xy=on  downsample_count=1  ovr_cals=on  ovr_actions=on  show_actions=off  action1_name=''  action1_cond=(None)  action2_name=''  action2_cond=(None)  action3_name=''  action3_cond=(None)  action4_name=''  action4_cond=(None)
  motohawk_fault_status1 : MotoHawk_lib/Fault Management Blocks/motohawk_fault_status  source=Lookup By Name  nam=[prefix 'RangeHigh']  status=Active
  motohawk_fault_status2 : MotoHawk_lib/Fault Management Blocks/motohawk_fault_status  source=Lookup By Name  nam=[prefix 'RangeHigh']  status=Suspected
  motohawk_fault_status3 : MotoHawk_lib/Fault Management Blocks/motohawk_fault_status  source=Lookup By Name  nam=[prefix 'RangeLow']  status=Suspected
  motohawk_fault_status4 : MotoHawk_lib/Fault Management Blocks/motohawk_fault_status  source=Lookup By Name  nam=[prefix 'RangeLow']  status=Active
  EngUnitsFilt : Outport  OutDataType=sfix(16)  OutScaling=2^0
  EngUnitsRaw : Outport  Port=2  OutDataType=sfix(16)  OutScaling=2^0
  wires:
  Logical Operator4/1 -> If/2, Logical Operator6/1
  Logical Operator1/1 -> Logical Operator5/2
  Logical Operator5/1 -> If/1
  Logical Operator6/1 -> Logical Operator5/1
  First Order Low Pass/1 -> Override/1
  motohawk_calibration3/1 -> If Action Subsystem1/1(In)
  Unit Delay1/1 -> If Action Subsystem/1(In)
  If/2 -> If Action Subsystem1/Action
  If Action Subsystem1/1(Out) -> Merge/3
  motohawk_fault_status4/1 -> Logical Operator4/2
  motohawk_fault_status1/1 -> Logical Operator4/1
  ZeroFullCal/1 -> Saturation/1
  If Action Subsystem/1(Out) -> Merge/2
  If Action Subsystem2/1(Out) -> Merge/1
  motohawk_fault_status3/1 -> Logical Operator1/2
  motohawk_fault_status2/1 -> Logical Operator1/1
  motohawk_calibration6/1 -> Relational Operator3/2
  motohawk_calibration1/1 -> Relational Operator2/2
  Relational Operator2/1 -> Logical Operator2/2
  Relational Operator3/1 -> Logical Operator3/2
  Logical Operator2/1 -> motohawk_fault_def2/1
  Logical Operator3/1 -> motohawk_fault_def3/1
  motohawk_data_read1/1 -> Logical Operator3/1, Logical Operator2/1
  Override/1 -> EngUnitsFilt/1, Final Value/1
  ADC/1 -> Data Type Conversion/1, From Analog Input/1
  Data Type Conversion/1 -> Relational Operator3/1, Relational Operator2/1, Mux/1
  If/1 -> If Action Subsystem/Action
  If/3 -> If Action Subsystem2/Action
  Merge/1 -> First Order Low Pass/1, EngUnitsRaw/1, Unit Delay1/1
  Mux/1 -> ZeroFullCal/1
  Saturation/1 -> "Unfiltered, Before Range Checking"/1, If Action Subsystem2/1(In)
  motohawk_calibration5/1 -> Mux/2
  motohawk_calibration4/1 -> Mux/3
